simulink subsystem "TRIAD"  (R2023b)
settings: Solver=VariableStepAuto  StartTime=0.0  StopTime=10.0  RelTol=1e-3
undefined symbols (not defined in the file): sensor_data
libraries: matrix_library x4
settings Model: Creator=pierb  LastModifiedBy=Pier Francesco

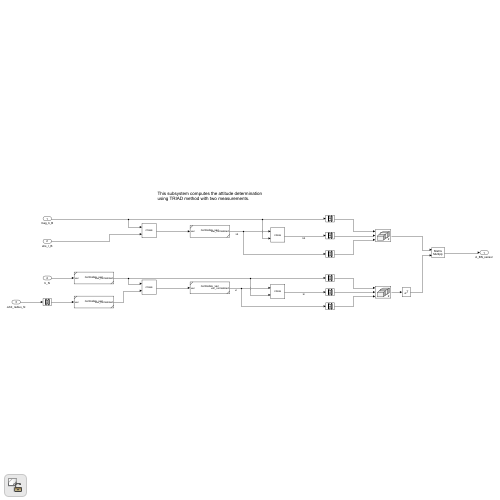
[thumbnail: Simulink's stored preview of the top-level diagram]
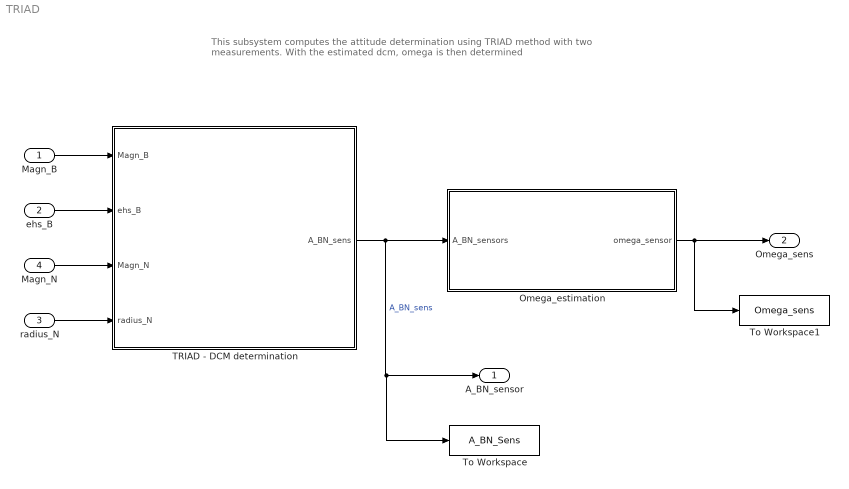
== system TRIAD ==
  note: This subsystem computes the attitude determination
      | using TRIAD method with two measurements.
      | With the estimated dcm, omega is then determined
  Magn_B : Inport
  ehs_B : Inport  Port=2
  radius_N : Inport  Port=3
  Magn_N : Inport  Port=4
  Omega_estimation : Subsystem
  TRIAD - DCM determination : Subsystem
  To Workspace : ToWorkspace  VariableName=A_BN_Sens  SampleTime=-1
  To Workspace1 : ToWorkspace  VariableName=Omega_sens  SampleTime=-1
  A_BN_sensor : Outport
  Omega_sens : Outport  Port=2
  wires:
  Magn_B/1 -> TRIAD - DCM determination/1(Magn_B)
  ehs_B/1 -> TRIAD - DCM determination/2(ehs_B)
  TRIAD - DCM determination/1(A_BN_sens) -> A_BN_sensor/1, To Workspace/1, Omega_estimation/1(A_BN_sensors)  "A_BN_sens"
  Magn_N/1 -> TRIAD - DCM determination/3(Magn_N)
  radius_N/1 -> TRIAD - DCM determination/4(radius_N)
  Omega_estimation/1(omega_sensor) -> Omega_sens/1, To Workspace1/1

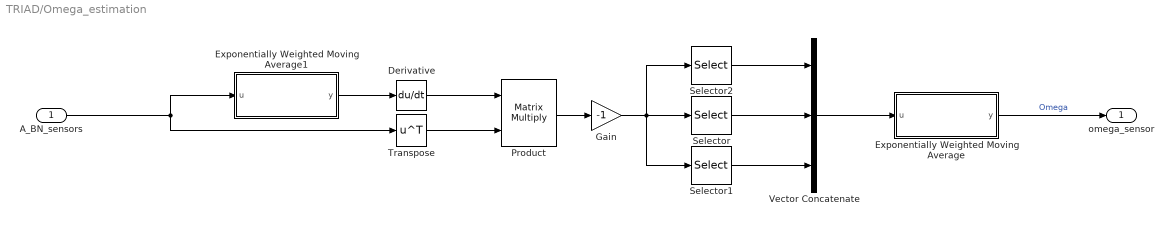
== system TRIAD/Omega_estimation ==
  A_BN_sensors : Inport
  Derivative : Derivative
  Exponentially Weighted Moving Average : Subsystem
  Exponentially Weighted Moving Average1 : Subsystem
  Gain : Gain  Gain=-1
  Product : Product  Multiplication=Matrix(*)
  Selector : Selector  NumberOfDimensions=2  InputPortWidth=3  IndexOptions=Index vector (dialog),Index vector (dialog)  Indices=1,3  OutputSizes=1,1
  Selector1 : Selector  NumberOfDimensions=2  InputPortWidth=3  IndexOptions=Index vector (dialog),Index vector (dialog)  Indices=2,1  OutputSizes=1,1
  Selector2 : Selector  NumberOfDimensions=2  InputPortWidth=3  IndexOptions=Index vector (dialog),Index vector (dialog)  Indices=3,2  OutputSizes=1,1
  Transpose : Math  Operator=transpose
  Vector Concatenate : Concatenate  NumInputs=3
  omega_sensor : Outport
  wires:
  Derivative/1 -> Product/1
  Transpose/1 -> Product/2
  Selector2/1 -> Vector Concatenate/1
  Exponentially Weighted Moving Average1/1(y) -> Derivative/1
  Gain/1 -> Selector/1, Selector2/1, Selector1/1
  Selector1/1 -> Vector Concatenate/3
  Selector/1 -> Vector Concatenate/2
  A_BN_sensors/1 -> Transpose/1, Exponentially Weighted Moving Average1/1(u)
  Exponentially Weighted Moving Average/1(y) -> omega_sensor/1  "Omega"
  Product/1 -> Gain/1
  Vector Concatenate/1 -> Exponentially Weighted Moving Average/1(u)

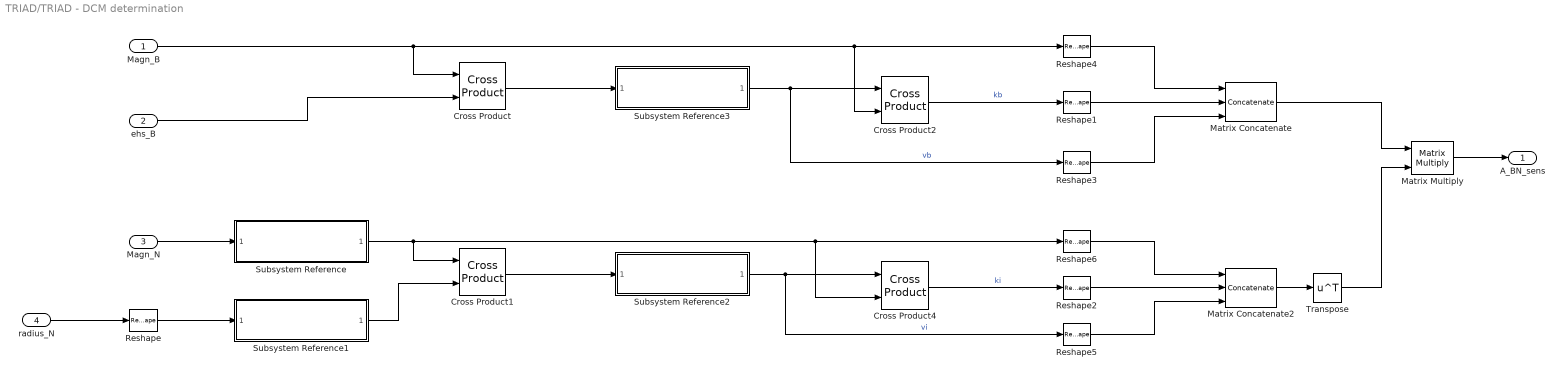
== system TRIAD/TRIAD - DCM determination ==
  Magn_B : Inport
  ehs_B : Inport  Port=2
  Magn_N : Inport  Port=3
  radius_N : Inport  Port=4
  Cross Product{,1..2,4} (4 alike) : matrix_library/Cross Product
  Matrix Concatenate : Concatenate  NumInputs=3  Mode=Multidimensional array  ConcatenateDimension=2
  Matrix Concatenate2 : Concatenate  NumInputs=3  Mode=Multidimensional array  ConcatenateDimension=2
  Matrix Multiply : Product  Multiplication=Matrix(*)
  Reshape{,1..6} (7 alike) : Reshape  OutputDimensionality=Column vector (2-D)
  Subsystem Reference{,1..3} (4 alike) : Subsystem  ReferencedSubsystem=normalize_vec
  Transpose : Math  Operator=transpose
  A_BN_sens : Outport
  wires:
  Reshape/1 -> Subsystem Reference1/1
  ehs_B/1 -> Cross Product/2
  Magn_N/1 -> Subsystem Reference/1
  Matrix Multiply/1 -> A_BN_sens/1
  Cross Product4/1 -> Reshape2/1  "ki"
  Cross Product/1 -> Subsystem Reference3/1
  Reshape5/1 -> Matrix Concatenate2/3
  Matrix Concatenate2/1 -> Transpose/1
  Reshape4/1 -> Matrix Concatenate/1
  Matrix Concatenate/1 -> Matrix Multiply/1
  Magn_B/1 -> Cross Product/1, Cross Product2/2, Reshape4/1
  Reshape6/1 -> Matrix Concatenate2/1
  Reshape2/1 -> Matrix Concatenate2/2
  Subsystem Reference1/1 -> Cross Product1/2
  Transpose/1 -> Matrix Multiply/2
  Reshape1/1 -> Matrix Concatenate/2
  Reshape3/1 -> Matrix Concatenate/3
  Subsystem Reference/1 -> Cross Product1/1, Reshape6/1, Cross Product4/2
  Cross Product2/1 -> Reshape1/1  "kb"
  Cross Product1/1 -> Subsystem Reference2/1
  radius_N/1 -> Reshape/1
  Subsystem Reference3/1 -> Reshape3/1, Cross Product2/1  "vb"
  Subsystem Reference2/1 -> Cross Product4/1, Reshape5/1  "vi"

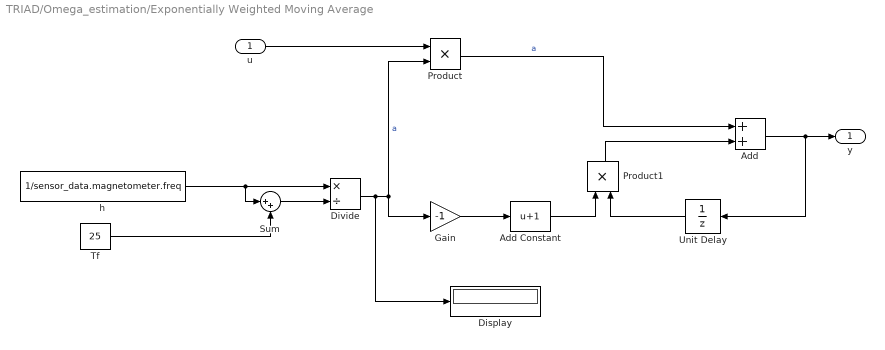
== system TRIAD/Omega_estimation/Exponentially Weighted Moving Average ==
  u : Inport
  Add : Sum
  Add Constant : Bias  Bias=1  SaturateOnIntegerOverflow=off
  Display : Display
  Divide : Product  Inputs=*/
  Gain : Gain  Gain=-1
  Product : Product  Inputs=**
  Product1 : Product
  Sum : Sum  Inputs=|++
  Tf : Constant  Value=25
  Unit Delay : UnitDelay  SampleTime=-1  HasFrameUpgradeWarning=on
  h : Constant  Value=1/sensor_data.magnetometer.freq
  y : Outport
  wires:
  Product1/1 -> Add/2
  Unit Delay/1 -> Product1/2
  Add Constant/1 -> Product1/1
  Gain/1 -> Add Constant/1
  Product/1 -> Add/1  "a"
  u/1 -> Product/1
  Divide/1 -> Gain/1, Product/2, Display/1  "a"
  Tf/1 -> Sum/2
  Sum/1 -> Divide/2
  h/1 -> Divide/1, Sum/1
  Add/1 -> y/1, Unit Delay/1

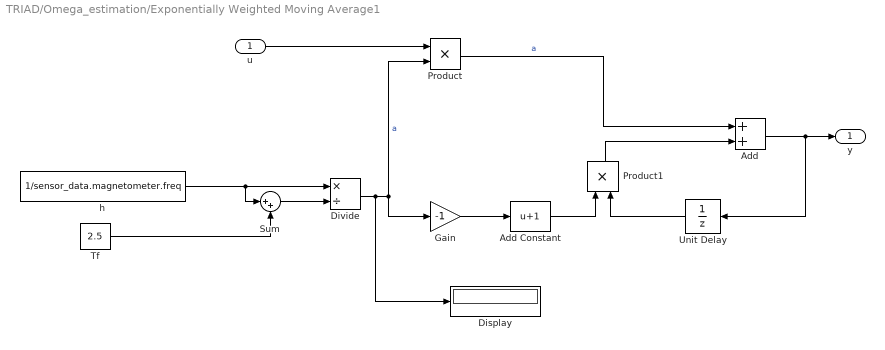
== system TRIAD/Omega_estimation/Exponentially Weighted Moving Average1 ==
  u : Inport
  Add : Sum
  Add Constant : Bias  Bias=1  SaturateOnIntegerOverflow=off
  Display : Display
  Divide : Product  Inputs=*/
  Gain : Gain  Gain=-1
  Product : Product  Inputs=**
  Product1 : Product
  Sum : Sum  Inputs=|++
  Tf : Constant  Value=2.5
  Unit Delay : UnitDelay  SampleTime=-1  HasFrameUpgradeWarning=on
  h : Constant  Value=1/sensor_data.magnetometer.freq
  y : Outport
  wires:
  Add/1 -> Unit Delay/1, y/1
  h/1 -> Sum/1, Divide/1
  Sum/1 -> Divide/2
  Tf/1 -> Sum/2
  Divide/1 -> Display/1, Product/2, Gain/1  "a"
  u/1 -> Product/1
  Product/1 -> Add/1  "a"
  Gain/1 -> Add Constant/1
  Add Constant/1 -> Product1/1
  Unit Delay/1 -> Product1/2
  Product1/1 -> Add/2
